simulink model "Furuta_Strecke"  (R2023b)
settings: Solver=VariableStepAuto  StartTime=0.0  StopTime=10  FixedStep=0.0001  RelTol=1e-3
values from neighbouring files (symbols this model uses):
  Acl = (A-B*K)    [Furuta_Parameter.m]
  alpha_0 = deg2rad(90)    [Furuta_Parameter.m]
  alpha_p0 = 0    [Furuta_Parameter.m]
  b1 = 0.0024    [Furuta_Parameter.m]
  b2 = 0.0024    [Furuta_Parameter.m]
  c1 = m1*lc1^2 + m2*l1^2 + J1 + J2z    (= 0.00790555064)    [Furuta_Parameter.m]
  c2 = m2*lc2^2 + J2x - J2z    (= 0.00427184272)    [Furuta_Parameter.m]
  c3 = m2*l1*lc2    (= 0.00426644308)    [Furuta_Parameter.m]
  c5 = m2*g*lc2    (= 0.193857372)    [Furuta_Parameter.m]
  k = 0.1285    [Furuta_Parameter.m]
  sigma = 0.069    [Furuta_Parameter.m]
  theta_0 = deg2rad(180)    [Furuta_Parameter.m]
  theta_p0 = 0    [Furuta_Parameter.m]
settings Model: Creator=dassow  LastModifiedBy=FrederikRittervonBae
settings SolverCC: AlgebraicLoopSolver=TrustRegion
settings DataIOCC: ReturnWorkspaceOutputs=off
settings DebuggingCC: UnconnectedInputMsg=warning  UnconnectedOutputMsg=warning  UnconnectedLineMsg=warning  ArithmeticOperatorsInVariantConditions=warning
settings ModelReferenceCC: EnableRefExpFcnMdlSchedulingChecks=on
settings SFSimCC: SimUseLocalCustomCode=off  CustomCodeUndefinedFunction=UseInterfaceOnly
settings RTWCC: RTWUseLocalCustomCode=off  DLArmComputeVersion=19.05

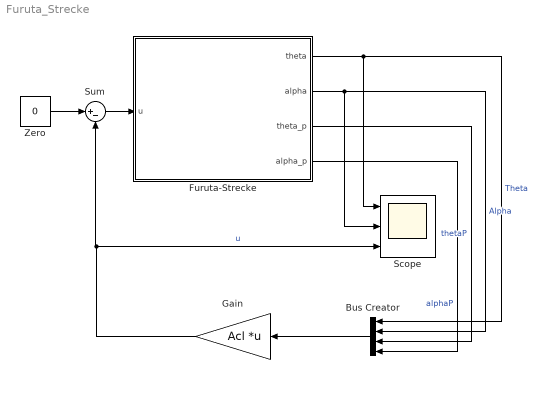
== system Furuta_Strecke ==
  Bus Creator : BusCreator  Inputs=4
  Furuta-Strecke : Subsystem
  Gain : Gain  Gain=Acl  Multiplication=Matrix(K*u) (u vector)
  Scope : Scope  NumInputPorts=3
  Sum : Sum  Inputs=|+-
  Zero : Constant  Value=0  OutDataTypeStr=Inherit: Inherit via back propagation
  wires:
  Furuta-Strecke/1(theta) -> Scope/1, Bus Creator/1  "Theta"
  Furuta-Strecke/2(alpha) -> Scope/2, Bus Creator/2  "Alpha"
  Gain/1 -> Sum/2, Scope/3  "u"
  Bus Creator/1 -> Gain/1
  Furuta-Strecke/3(theta_p) -> Bus Creator/3  "thetaP"
  Furuta-Strecke/4(alpha_p) -> Bus Creator/4  "alphaP"
  Zero/1 -> Sum/1
  Sum/1 -> Furuta-Strecke/1(u)

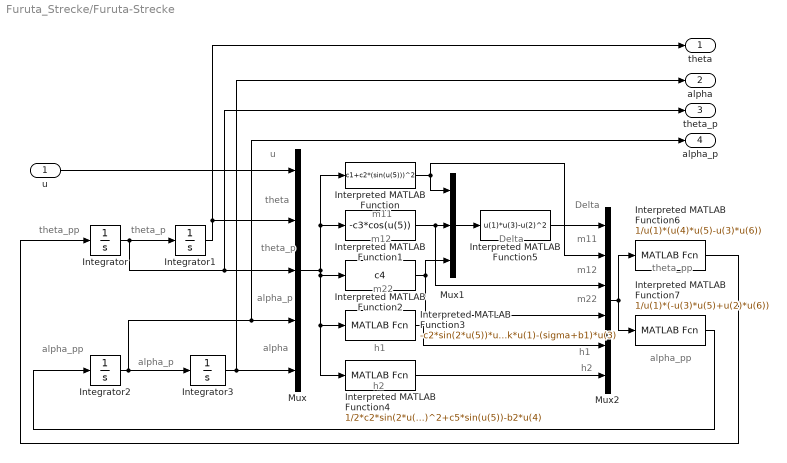
== system Furuta_Strecke/Furuta-Strecke ==
  note: alpha_pp
  note: alpha_pp
  note: theta_pp
  note: h2
  note: h1
  note: m22
  note: m12
  note: Delta
  note: m11
  note: Delta
  note: h2
  note: h1
  note: m22
  note: m12
  note: m11
  note: alpha
  note: alpha_p
  note: theta_pp
  note: theta_p
  note: theta
  note: u
  note: theta_p
  note: alpha_p
  u : Inport
  Integrator : Integrator  InitialCondition=theta_p0
  "Integrator1 " : Integrator  InitialCondition=theta_0
  Integrator2 : Integrator  InitialCondition=alpha_p0
  "Integrator3 " : Integrator  InitialCondition=alpha_0
  Interpreted MATLAB Function : MATLABFcn  MATLABFcn=c1+c2*(sin(u(5)))^2  OutputDimensions=1
  Interpreted MATLAB Function1 : MATLABFcn  MATLABFcn=-c3*cos(u(5))  OutputDimensions=1
  Interpreted MATLAB Function2 : MATLABFcn  MATLABFcn=c4  OutputDimensions=1
  Interpreted MATLAB Function3 : MATLABFcn  MATLABFcn=-c2*sin(2*u(5))*u(4)*u(3) - c3*sin(u(5))*u(4)^2+k*u(1)-(sigma+b1)*u(3)  OutputDimensions=1
  Interpreted MATLAB Function4 : MATLABFcn  MATLABFcn=1/2*c2*sin(2*u(5))*u(3)^2+c5*sin(u(5))-b2*u(4)  OutputDimensions=1
  Interpreted MATLAB Function5 : MATLABFcn  MATLABFcn=u(1)*u(3)-u(2)^2  OutputDimensions=1
  Interpreted MATLAB Function6 : MATLABFcn  MATLABFcn=1/u(1)*(u(4)*u(5)-u(3)*u(6))  OutputDimensions=1
  Interpreted MATLAB Function7 : MATLABFcn  MATLABFcn=1/u(1)*(-u(3)*u(5)+u(2)*u(6))  OutputDimensions=1
  Mux : Mux  Inputs=5
  Mux1 : Mux  Inputs=3
  Mux2 : Mux  Inputs=6
  theta : Outport
  alpha : Outport  Port=2
  theta_p : Outport  Port=3
  alpha_p : Outport  Port=4
  wires:
  Interpreted MATLAB Function4/1 -> Mux2/6
  Interpreted MATLAB Function6/1 -> Integrator/1
  Interpreted MATLAB Function5/1 -> Mux2/1
  "Integrator3 "/1 -> alpha/1, Mux/5
  Interpreted MATLAB Function2/1 -> Mux2/4, Mux1/3
  Interpreted MATLAB Function3/1 -> Mux2/5
  Interpreted MATLAB Function7/1 -> Integrator2/1
  u/1 -> Mux/1
  Mux1/1 -> Interpreted MATLAB Function5/1
  Integrator/1 -> "Integrator1 "/1, theta_p/1, Mux/3
  Interpreted MATLAB Function1/1 -> Mux2/3, Mux1/2
  "Integrator1 "/1 -> theta/1, Mux/2
  Mux/1 -> Interpreted MATLAB Function4/1, Interpreted MATLAB Function3/1, Interpreted MATLAB Function2/1, Interpreted MATLAB Function/1, Interpreted MATLAB Function1/1
  Interpreted MATLAB Function/1 -> Mux2/2, Mux1/1
  Mux2/1 -> Interpreted MATLAB Function7/1, Interpreted MATLAB Function6/1
  Integrator2/1 -> Mux/4, alpha_p/1, "Integrator3 "/1
